simulink subsystem "ThreeAxesSignals"  (R2021a)
settings: Solver=VariableStepAuto  StartTime=0.0  StopTime=10.0  RelTol=1e-3
undefined symbols (not defined in the file): pitch, roll, t0x, t0y, t0z, tfx, tfy, tfz, yaw
libraries: simulink x6
settings Model: Creator=Laura  LastModifiedBy=Laura

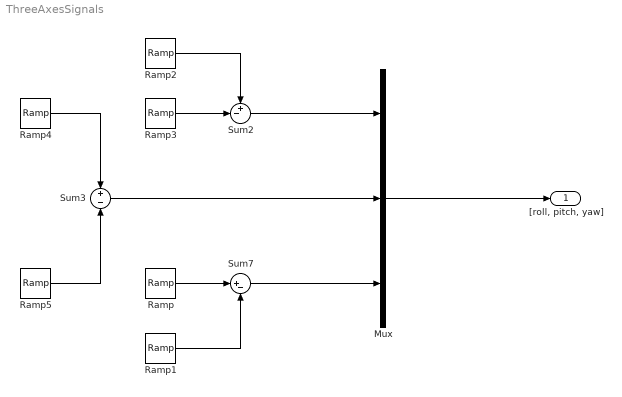
== system ThreeAxesSignals ==
  Mux : Mux  Inputs=3
  Ramp : simulink/Sources/Ramp  slope=yaw/(tfz - t0z)  start=t0z  InitialOutput=0
  Ramp1 : simulink/Sources/Ramp  slope=yaw/(tfz - t0z)  start=tfz  InitialOutput=0
  Ramp2 : simulink/Sources/Ramp  slope=roll/(tfx - t0x)  start=t0x  InitialOutput=0
  Ramp3 : simulink/Sources/Ramp  slope=roll/(tfx - t0x)  start=tfx  InitialOutput=0
  Ramp4 : simulink/Sources/Ramp  slope=pitch/(tfy - t0y)  start=t0y  InitialOutput=0
  Ramp5 : simulink/Sources/Ramp  slope=pitch/(tfy - t0y)  start=tfy  InitialOutput=0
  Sum2 : Sum  Inputs=+-|
  Sum3 : Sum  Inputs=+-
  Sum7 : Sum  Inputs=|+-
  "[roll, pitch, yaw]" : Outport
  wires:
  Ramp4/1 -> Sum3/1
  Ramp/1 -> Sum7/1
  Ramp5/1 -> Sum3/2
  Ramp2/1 -> Sum2/1
  Ramp3/1 -> Sum2/2
  Ramp1/1 -> Sum7/2
  Sum2/1 -> Mux/1
  Sum3/1 -> Mux/2
  Sum7/1 -> Mux/3
  Mux/1 -> "[roll, pitch, yaw]"/1
